simulink model "Osc1CarrierTestHarness"  (R2024a)
settings: Solver=VariableStepAuto  StartTime=0.0  StopTime=10.0  RelTol=1e-3
model workspace (MAT data in the model file):
  amp_max = 1
  amp_min = -1
  max_midi_data = Simulink.Parameter
  max_midi_data.Value = 127
  max_midi_data.Complexity = 'real'
  max_midi_data.Dimensions = [1 1]
  max_midi_data.DataType = 'uint8'
  osc_sampling_freq = Simulink.Parameter
  osc_sampling_freq.Value = 48000
  osc_sampling_freq.Complexity = 'real'
  osc_sampling_freq.Dimensions = [1 1]
  osc_sampling_freq.DataType = 'auto'
  wave_len = Simulink.Parameter
  wave_len.Value = 256
  wave_len.Complexity = 'real'
  wave_len.Dimensions = [1 1]
  wave_len.DataType = 'auto'
  xtones = Simulink.Parameter
  xtones.Value = 120
  xtones.Complexity = 'real'
  xtones.Dimensions = [1 1]
  xtones.Description = 'Number of "x" tones in an octave
    | 
    | By default, an octave is 12 semi-tones.
    | To detune a frequency more finely, we divide an octave in a number of xtones, which should be a multiple of 12: x xtones is 12 semi-tones.
    | '
  xtones.DataType = 'int16'
settings Model: Creator=dfurodet  LastModifiedBy=dfurodet
settings DebuggingCC: UnderspecifiedInitializationDetection=Classic  MergeDetectMultiDrivingBlocksExec=none
settings ModelReferenceCC: PropagateSignalLabelsOutOfModel=off

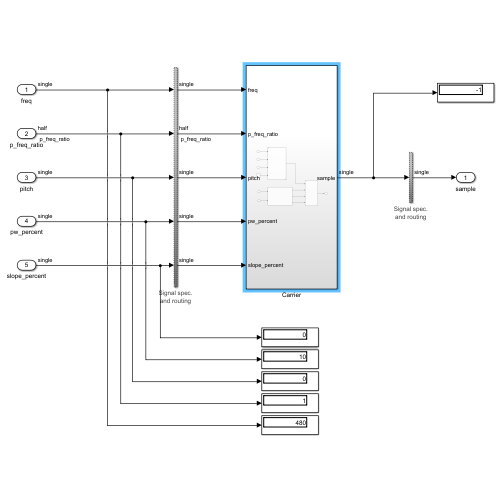
[thumbnail: Simulink's stored preview of the top-level diagram]
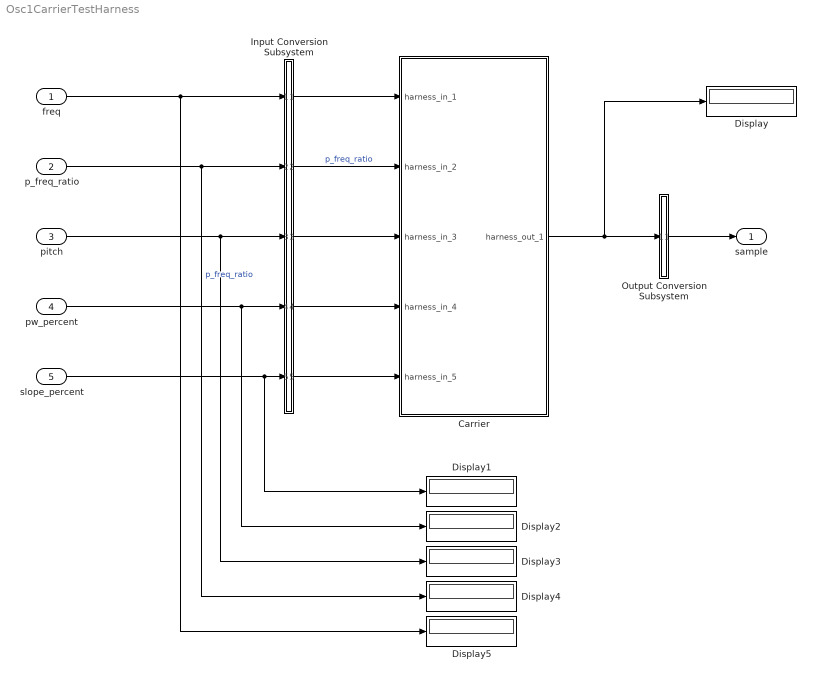
== system Osc1CarrierTestHarness ==
  freq : Inport  OutDataTypeStr=single  PortDimensions=[1]  SampleTime=1
  p_freq_ratio : Inport  Port=2  OutDataTypeStr=half  PortDimensions=[1]  SampleTime=[-1, 0]
  pitch : Inport  Port=3  OutDataTypeStr=single  PortDimensions=[1]  SampleTime=1
  pw_percent : Inport  Port=4  OutDataTypeStr=single  PortDimensions=[1]  SampleTime=1
  slope_percent : Inport  Port=5  OutDataTypeStr=single  PortDimensions=[1]  SampleTime=1
  Carrier : Subsystem  Tag=__SL_testing_harness_stub_
  Display{,1..5} (6 alike) : Display
  Input Conversion Subsystem : Subsystem  Tag=__SLT_ICS__  Description=|
      | Signal spec.
      | and routing
      settings: AttributesFormatString=%<Description>
  Output Conversion Subsystem : Subsystem  Tag=__SLT_OCS__  Description=|
      | Signal spec.
      | and routing
      settings: AttributesFormatString=%<Description>
  sample : Outport
  wires:
  freq/1 -> Display5/1, Input Conversion Subsystem/1(Inport_1)
  p_freq_ratio/1 -> Display4/1, Input Conversion Subsystem/2(Inport_2)  "p_freq_ratio"
  pitch/1 -> Display3/1, Input Conversion Subsystem/3(Inport_3)
  pw_percent/1 -> Display2/1, Input Conversion Subsystem/4(Inport_4)
  slope_percent/1 -> Input Conversion Subsystem/5(Inport_5), Display1/1
  Output Conversion Subsystem/1(Outport_1) -> sample/1
  Input Conversion Subsystem/1(Outport_1) -> Carrier/1(harness_in_1)
  Input Conversion Subsystem/2(Outport_2) -> Carrier/2(harness_in_2)  "p_freq_ratio"
  Input Conversion Subsystem/3(Outport_3) -> Carrier/3(harness_in_3)
  Input Conversion Subsystem/4(Outport_4) -> Carrier/4(harness_in_4)
  Input Conversion Subsystem/5(Outport_5) -> Carrier/5(harness_in_5)
  Carrier/1(harness_out_1) -> Display/1, Output Conversion Subsystem/1(Inport_1)

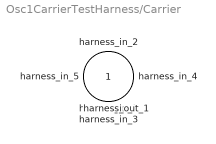
== system Osc1CarrierTestHarness/Carrier ==
  harness_in_1 : Inport
  harness_in_2 : Inport  Port=2
  harness_in_3 : Inport  Port=3
  harness_in_4 : Inport  Port=4
  harness_in_5 : Inport  Port=5
  harness_out_1 : Outport

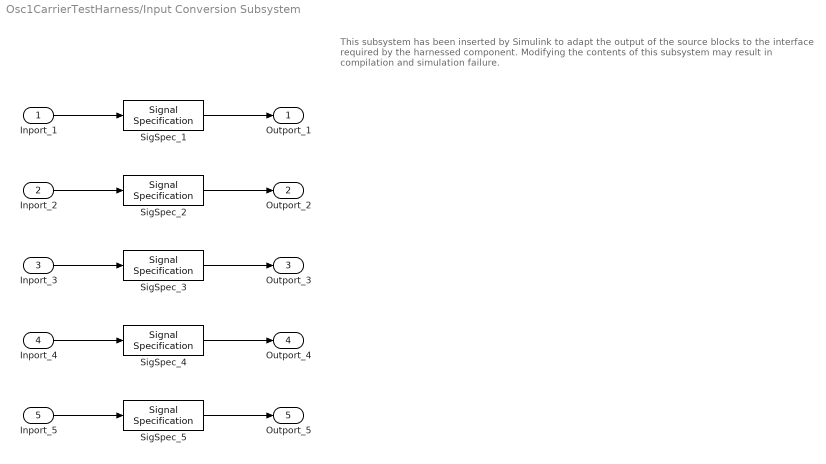
== system Osc1CarrierTestHarness/Input Conversion Subsystem ==
  note: This subsystem has been inserted by Simulink to adapt the output of the source blocks to the interface required by the harnessed component.
      |  Modifying the contents of this subsystem may result in compilation and simulation failure.
  Inport_1 : Inport
  Inport_2 : Inport  Port=2
  Inport_3 : Inport  Port=3
  Inport_4 : Inport  Port=4
  Inport_5 : Inport  Port=5
  SigSpec_{1,3..5} (4 alike) : SignalSpecification  OutDataTypeStr=single  Dimensions=[1]  SampleTime=1
  SigSpec_2 : SignalSpecification  OutDataTypeStr=half  Dimensions=[1]  SampleTime=[-1, 0]
  Outport_1 : Outport
  Outport_2 : Outport  Port=2
  Outport_3 : Outport  Port=3
  Outport_4 : Outport  Port=4
  Outport_5 : Outport  Port=5
  wires:
  SigSpec_1/1 -> Outport_1/1
  Inport_1/1 -> SigSpec_1/1
  SigSpec_2/1 -> Outport_2/1
  Inport_2/1 -> SigSpec_2/1
  SigSpec_3/1 -> Outport_3/1
  Inport_3/1 -> SigSpec_3/1
  SigSpec_4/1 -> Outport_4/1
  Inport_4/1 -> SigSpec_4/1
  SigSpec_5/1 -> Outport_5/1
  Inport_5/1 -> SigSpec_5/1

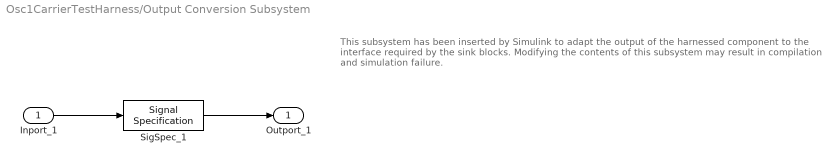
== system Osc1CarrierTestHarness/Output Conversion Subsystem ==
  note: This subsystem has been inserted by Simulink to adapt the output of the harnessed component to the interface required by the sink blocks.
      |  Modifying the contents of this subsystem may result in compilation and simulation failure.
  Inport_1 : Inport
  SigSpec_1 : SignalSpecification  OutDataTypeStr=single  Dimensions=[1]  SampleTime=1
  Outport_1 : Outport
  wires:
  Inport_1/1 -> SigSpec_1/1
  SigSpec_1/1 -> Outport_1/1
